simulink subsystem "harmonicFeatures"  (R2020b)
settings: Solver=VariableStepAuto  StartTime=0.0  StopTime=10.0  RelTol=1e-3
undefined symbols (not defined in the file or in its folder): params
libraries: dspstat3 x1
settings Model: Creator=trevor  LastModifiedBy=trevor

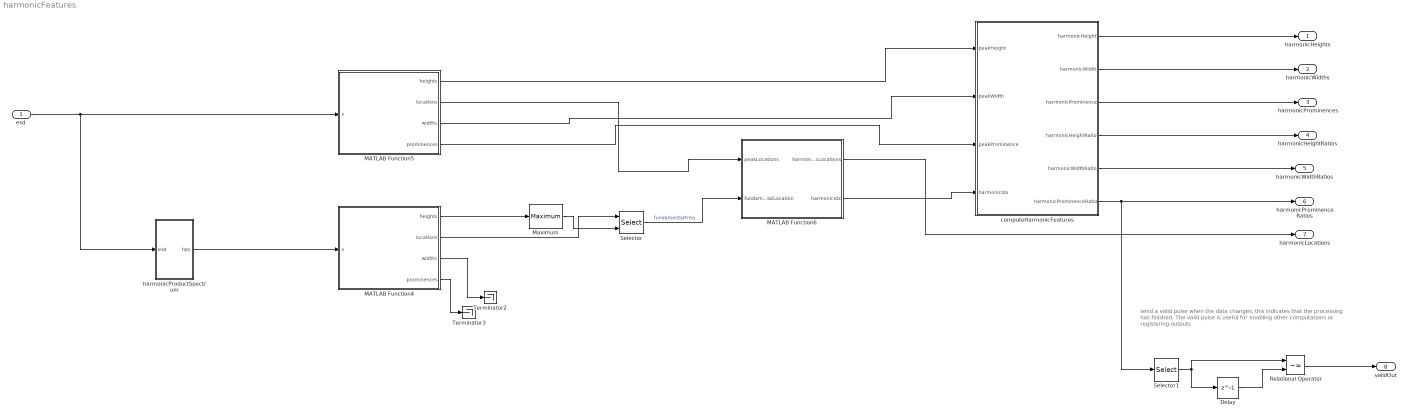
== system harmonicFeatures ==
  note: send a valid pulse when the data changes;
      | this indicates that the processing has finished.
      | The valid pulse is useful for enabling other
      | computations or registering outputs
  esd : Inport
  Delay : Delay  DelayLength=1
  MATLAB Function4 : MATLAB Function  TreatAsAtomicUnit=on
  MATLAB Function5 : MATLAB Function  TreatAsAtomicUnit=on
  MATLAB Function6 : MATLAB Function  TreatAsAtomicUnit=on
  Maximum : dspstat3/Maximum  operation=maximum  fcn=Index  indexBase=One  operateOver=Each row  Dimension=1  InputProcessing=Columns as channels (frame based)  reset=None  roiEnable=off  roiType=Rectangles  roiPortion=Entire ROI  roiOutput=Individual statistics for each ROI  roiFlag=off  roundingMode=Floor  overflowMode=off  accumDataTypeStr=Inherit: Same as product output  accumLastDataTypeStr=Inherit: Same as product output
  Relational Operator : RelationalOperator  Operator=~=  OutDataTypeStr=boolean  RndMeth=Simplest
  Selector : Selector  InputPortWidth=85  IndexOptions=Index vector (port)  Indices=[1 3]  OutputSizes=1
  Selector1 : Selector  InputPortWidth=3  IndexOptions=Index vector (dialog)  Indices=1  OutputSizes=1
  Terminator2 : Terminator
  Terminator3 : Terminator
  computeHarmonicFeatures : Subsystem
  harmonicProductSpectrum : Subsystem
  harmonicHeights : Outport
  harmonicWidths : Outport  Port=2
  harmonicProminences : Outport  Port=3
  harmonicHeightRatios : Outport  Port=4
  harmonicWidthRatios : Outport  Port=5
  harmonicProminenceRatios : Outport  Port=6
  harmonicLocations : Outport  Port=7
  validOut : Outport  Port=8
  wires:
  Selector1/1 -> Delay/1, Relational Operator/1
  Delay/1 -> Relational Operator/2
  Relational Operator/1 -> validOut/1
  Maximum/1 -> Selector/2
  MATLAB Function4/1(heights) -> Maximum/1
  harmonicProductSpectrum/1(hps) -> MATLAB Function4/1(x)
  MATLAB Function4/4(prominences) -> Terminator3/1
  MATLAB Function4/3(widths) -> Terminator2/1
  MATLAB Function4/2(locations) -> Selector/1
  esd/1 -> harmonicProductSpectrum/1(esd), MATLAB Function5/1(x)
  computeHarmonicFeatures/6(harmonicProminenceRatio) -> Selector1/1, harmonicProminenceRatios/1
  computeHarmonicFeatures/1(harmonicHeight) -> harmonicHeights/1
  computeHarmonicFeatures/2(harmonicWidth) -> harmonicWidths/1
  computeHarmonicFeatures/3(harmonicProminence) -> harmonicProminences/1
  computeHarmonicFeatures/4(harmonicHeightRatio) -> harmonicHeightRatios/1
  computeHarmonicFeatures/5(harmonicWidthRatio) -> harmonicWidthRatios/1
  MATLAB Function5/1(heights) -> computeHarmonicFeatures/1(peakHeight)
  MATLAB Function5/3(widths) -> computeHarmonicFeatures/2(peakWidth)
  MATLAB Function5/4(prominences) -> computeHarmonicFeatures/3(peakProminence)
  MATLAB Function5/2(locations) -> MATLAB Function6/1(peakLocations)
  Selector/1 -> MATLAB Function6/2(fundamentalLocation)  "fundamentalFreq"
  MATLAB Function6/1(harmonicLocations) -> harmonicLocations/1
  MATLAB Function6/2(harmonicIdx) -> computeHarmonicFeatures/4(harmonicIdx)

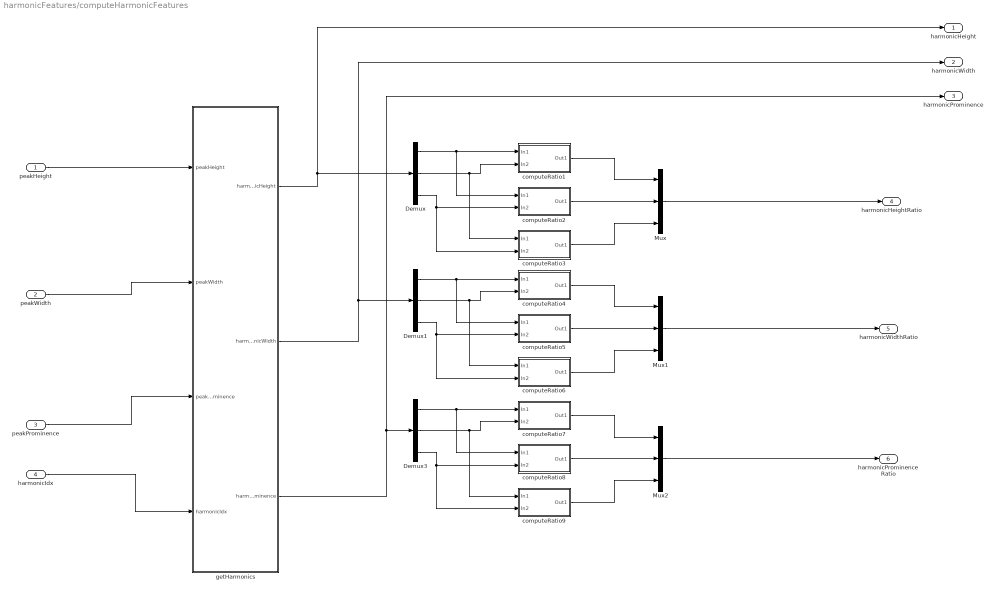
== system harmonicFeatures/computeHarmonicFeatures ==
  peakHeight : Inport
  peakWidth : Inport  Port=2
  peakProminence : Inport  Port=3
  harmonicIdx : Inport  Port=4
  Demux : Demux  Outputs=3
  Demux1 : Demux  Outputs=3
  Demux3 : Demux  Outputs=3
  Mux : Mux  Inputs=3
  Mux1 : Mux  Inputs=3
  Mux2 : Mux  Inputs=3
  computeRatio1 : Subsystem
  computeRatio2 : Subsystem
  computeRatio3 : Subsystem
  computeRatio4 : Subsystem
  computeRatio5 : Subsystem
  computeRatio6 : Subsystem
  computeRatio7 : Subsystem
  computeRatio8 : Subsystem
  computeRatio9 : Subsystem
  getHarmonics : Subsystem
  harmonicHeight : Outport
  harmonicWidth : Outport  Port=2
  harmonicProminence : Outport  Port=3
  harmonicHeightRatio : Outport  Port=4
  harmonicWidthRatio : Outport  Port=5
  harmonicProminenceRatio : Outport  Port=6
  wires:
  harmonicIdx/1 -> getHarmonics/4(harmonicIdx)
  peakProminence/1 -> getHarmonics/3(peakProminence)
  peakWidth/1 -> getHarmonics/2(peakWidth)
  peakHeight/1 -> getHarmonics/1(peakHeight)
  getHarmonics/2(harmonicWidth) -> Demux1/1, harmonicWidth/1
  getHarmonics/1(harmonicHeight) -> Demux/1, harmonicHeight/1
  getHarmonics/3(harmonicProminence) -> Demux3/1, harmonicProminence/1
  computeRatio9/1(Out1) -> Mux2/3
  computeRatio8/1(Out1) -> Mux2/2
  computeRatio7/1(Out1) -> Mux2/1
  computeRatio6/1(Out1) -> Mux1/3
  computeRatio4/1(Out1) -> Mux1/1
  computeRatio5/1(Out1) -> Mux1/2
  computeRatio3/1(Out1) -> Mux/3
  computeRatio1/1(Out1) -> Mux/1
  computeRatio2/1(Out1) -> Mux/2
  Demux3/2 -> computeRatio7/2(In2), computeRatio9/1(In1)
  Demux3/3 -> computeRatio8/2(In2), computeRatio9/2(In2)
  Demux3/1 -> computeRatio7/1(In1), computeRatio8/1(In1)
  Demux1/2 -> computeRatio4/2(In2), computeRatio6/1(In1)
  Demux1/3 -> computeRatio5/2(In2), computeRatio6/2(In2)
  Demux1/1 -> computeRatio4/1(In1), computeRatio5/1(In1)
  Demux/3 -> computeRatio2/2(In2), computeRatio3/2(In2)
  Demux/2 -> computeRatio1/2(In2), computeRatio3/1(In1)
  Demux/1 -> computeRatio1/1(In1), computeRatio2/1(In1)
  Mux/1 -> harmonicHeightRatio/1
  Mux1/1 -> harmonicWidthRatio/1
  Mux2/1 -> harmonicProminenceRatio/1

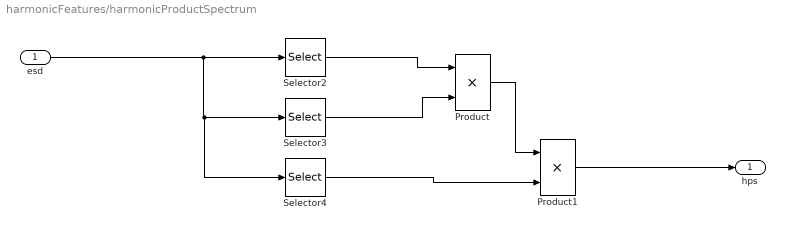
== system harmonicFeatures/harmonicProductSpectrum ==
  esd : Inport
  Product : Product  OutMin=0  OutMax=1
  Product1 : Product  OutDataTypeStr=Inherit: Same as first input
  Selector2 : Selector  InputPortWidth=512  IndexOptions=Index vector (dialog)  Indices=[1:1:170]  OutputSizes=1
  Selector3 : Selector  InputPortWidth=512  IndexOptions=Index vector (dialog)  Indices=[1:2:2*170]  OutputSizes=1
  Selector4 : Selector  InputPortWidth=512  IndexOptions=Index vector (dialog)  Indices=[1:3:3*170]  OutputSizes=1
  hps : Outport
  wires:
  Selector2/1 -> Product/1
  Product/1 -> Product1/1
  Selector4/1 -> Product1/2
  Product1/1 -> hps/1
  esd/1 -> Selector2/1, Selector3/1, Selector4/1
  Selector3/1 -> Product/2

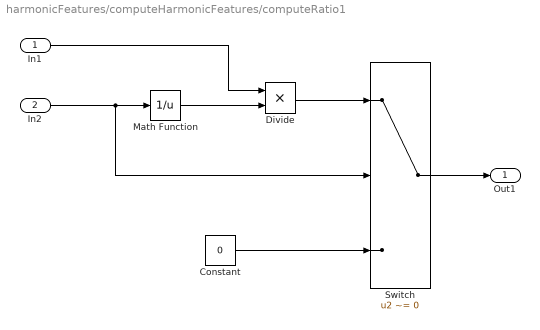
== system harmonicFeatures/computeHarmonicFeatures/computeRatio1 ==
  In1 : Inport
  In2 : Inport  Port=2
  Constant : Constant  Value=0  OutDataTypeStr=Inherit: Inherit via back propagation  SampleTime=params.systemClockPeriod
  Divide : Product  Inputs=**  OutDataTypeStr=Inherit: Keep MSB
  Math Function : Math  Operator=reciprocal  RndMeth=Zero  SaturateOnIntegerOverflow=on  OutDataTypeStr=Inherit: Inherit via internal rule
  Switch : Switch  Criteria=u2 ~= 0
  Out1 : Outport
  wires:
  Math Function/1 -> Divide/2
  Constant/1 -> Switch/3
  In2/1 -> Math Function/1, Switch/2
  Switch/1 -> Out1/1
  Divide/1 -> Switch/1
  In1/1 -> Divide/1

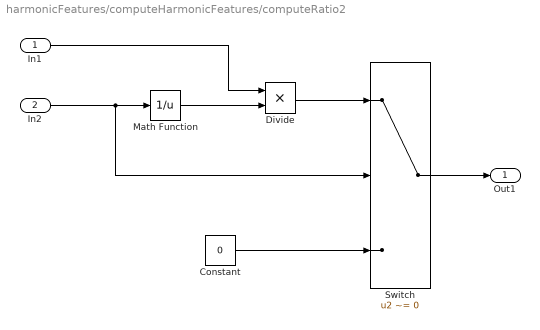
== system harmonicFeatures/computeHarmonicFeatures/computeRatio2 ==
  In1 : Inport
  In2 : Inport  Port=2
  Constant : Constant  Value=0  OutDataTypeStr=Inherit: Inherit via back propagation  SampleTime=params.systemClockPeriod
  Divide : Product  Inputs=**  OutDataTypeStr=Inherit: Keep MSB
  Math Function : Math  Operator=reciprocal  RndMeth=Zero  SaturateOnIntegerOverflow=on  OutDataTypeStr=Inherit: Inherit via internal rule
  Switch : Switch  Criteria=u2 ~= 0
  Out1 : Outport
  wires:
  Math Function/1 -> Divide/2
  Constant/1 -> Switch/3
  In2/1 -> Math Function/1, Switch/2
  Switch/1 -> Out1/1
  Divide/1 -> Switch/1
  In1/1 -> Divide/1

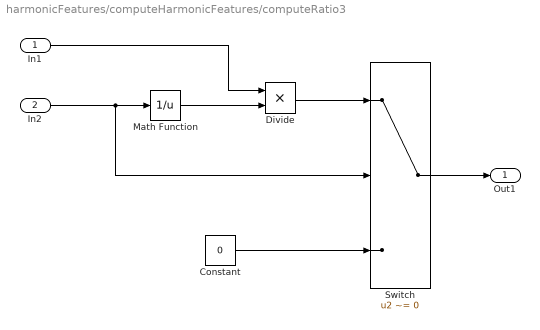
== system harmonicFeatures/computeHarmonicFeatures/computeRatio3 ==
  In1 : Inport
  In2 : Inport  Port=2
  Constant : Constant  Value=0  OutDataTypeStr=Inherit: Inherit via back propagation  SampleTime=params.systemClockPeriod
  Divide : Product  Inputs=**  OutDataTypeStr=Inherit: Keep MSB
  Math Function : Math  Operator=reciprocal  RndMeth=Zero  SaturateOnIntegerOverflow=on  OutDataTypeStr=Inherit: Inherit via internal rule
  Switch : Switch  Criteria=u2 ~= 0
  Out1 : Outport
  wires:
  Math Function/1 -> Divide/2
  Constant/1 -> Switch/3
  In2/1 -> Math Function/1, Switch/2
  Switch/1 -> Out1/1
  Divide/1 -> Switch/1
  In1/1 -> Divide/1

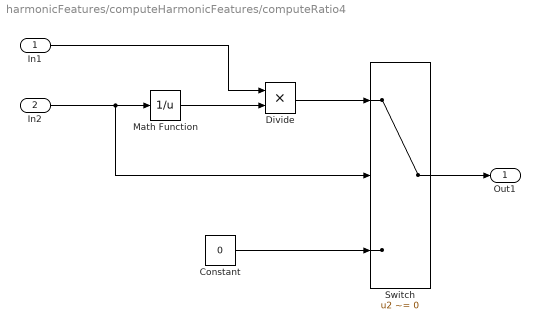
== system harmonicFeatures/computeHarmonicFeatures/computeRatio4 ==
  In1 : Inport
  In2 : Inport  Port=2
  Constant : Constant  Value=0  OutDataTypeStr=Inherit: Inherit via back propagation  SampleTime=params.systemClockPeriod
  Divide : Product  Inputs=**  OutDataTypeStr=Inherit: Keep MSB
  Math Function : Math  Operator=reciprocal  RndMeth=Zero  SaturateOnIntegerOverflow=on  OutDataTypeStr=Inherit: Inherit via internal rule
  Switch : Switch  Criteria=u2 ~= 0
  Out1 : Outport
  wires:
  Math Function/1 -> Divide/2
  Constant/1 -> Switch/3
  In2/1 -> Math Function/1, Switch/2
  Switch/1 -> Out1/1
  Divide/1 -> Switch/1
  In1/1 -> Divide/1

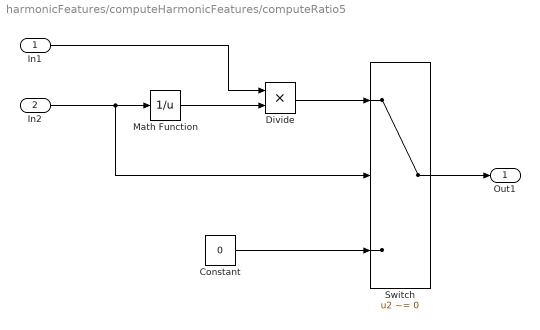
== system harmonicFeatures/computeHarmonicFeatures/computeRatio5 ==
  In1 : Inport
  In2 : Inport  Port=2
  Constant : Constant  Value=0  OutDataTypeStr=Inherit: Inherit via back propagation  SampleTime=params.systemClockPeriod
  Divide : Product  Inputs=**  OutDataTypeStr=Inherit: Keep MSB
  Math Function : Math  Operator=reciprocal  RndMeth=Zero  SaturateOnIntegerOverflow=on  OutDataTypeStr=Inherit: Inherit via internal rule
  Switch : Switch  Criteria=u2 ~= 0
  Out1 : Outport
  wires:
  Math Function/1 -> Divide/2
  Constant/1 -> Switch/3
  In2/1 -> Math Function/1, Switch/2
  Switch/1 -> Out1/1
  Divide/1 -> Switch/1
  In1/1 -> Divide/1

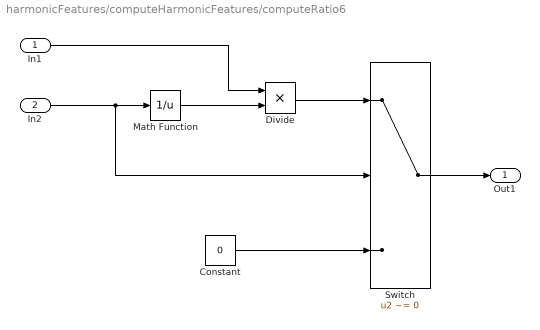
== system harmonicFeatures/computeHarmonicFeatures/computeRatio6 ==
  In1 : Inport
  In2 : Inport  Port=2
  Constant : Constant  Value=0  OutDataTypeStr=Inherit: Inherit via back propagation  SampleTime=params.systemClockPeriod
  Divide : Product  Inputs=**  OutDataTypeStr=Inherit: Keep MSB
  Math Function : Math  Operator=reciprocal  RndMeth=Zero  SaturateOnIntegerOverflow=on  OutDataTypeStr=Inherit: Inherit via internal rule
  Switch : Switch  Criteria=u2 ~= 0
  Out1 : Outport
  wires:
  Math Function/1 -> Divide/2
  Constant/1 -> Switch/3
  In2/1 -> Math Function/1, Switch/2
  Switch/1 -> Out1/1
  Divide/1 -> Switch/1
  In1/1 -> Divide/1

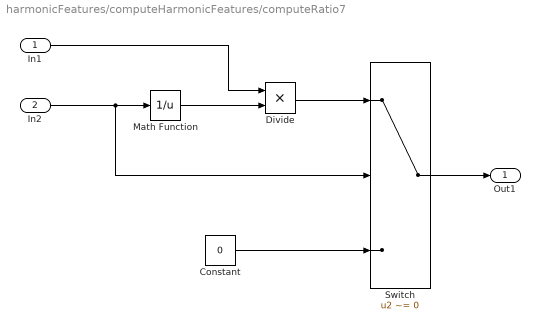
== system harmonicFeatures/computeHarmonicFeatures/computeRatio7 ==
  In1 : Inport
  In2 : Inport  Port=2
  Constant : Constant  Value=0  OutDataTypeStr=Inherit: Inherit via back propagation  SampleTime=params.systemClockPeriod
  Divide : Product  Inputs=**  OutDataTypeStr=Inherit: Keep MSB
  Math Function : Math  Operator=reciprocal  RndMeth=Zero  SaturateOnIntegerOverflow=on  OutDataTypeStr=Inherit: Inherit via internal rule
  Switch : Switch  Criteria=u2 ~= 0
  Out1 : Outport
  wires:
  Math Function/1 -> Divide/2
  Constant/1 -> Switch/3
  In2/1 -> Math Function/1, Switch/2
  Switch/1 -> Out1/1
  Divide/1 -> Switch/1
  In1/1 -> Divide/1

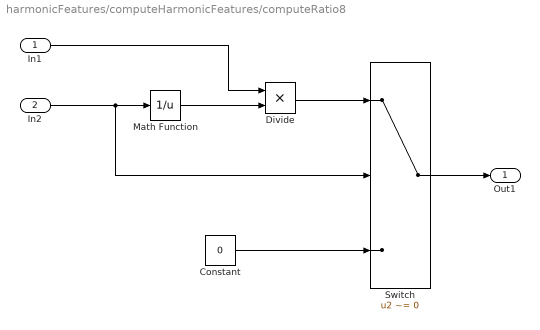
== system harmonicFeatures/computeHarmonicFeatures/computeRatio8 ==
  In1 : Inport
  In2 : Inport  Port=2
  Constant : Constant  Value=0  OutDataTypeStr=Inherit: Inherit via back propagation  SampleTime=params.systemClockPeriod
  Divide : Product  Inputs=**  OutDataTypeStr=Inherit: Keep MSB
  Math Function : Math  Operator=reciprocal  RndMeth=Zero  SaturateOnIntegerOverflow=on  OutDataTypeStr=Inherit: Inherit via internal rule
  Switch : Switch  Criteria=u2 ~= 0
  Out1 : Outport
  wires:
  Math Function/1 -> Divide/2
  Constant/1 -> Switch/3
  In2/1 -> Math Function/1, Switch/2
  Switch/1 -> Out1/1
  Divide/1 -> Switch/1
  In1/1 -> Divide/1

== system harmonicFeatures/computeHarmonicFeatures/computeRatio9 ==
  In1 : Inport
  In2 : Inport  Port=2
  Constant : Constant  Value=0  OutDataTypeStr=Inherit: Inherit via back propagation  SampleTime=params.systemClockPeriod
  Divide : Product  Inputs=**  OutDataTypeStr=Inherit: Keep MSB
  Math Function : Math  Operator=reciprocal  RndMeth=Zero  SaturateOnIntegerOverflow=on  OutDataTypeStr=Inherit: Inherit via internal rule
  Switch : Switch  Criteria=u2 ~= 0
  Out1 : Outport
  wires:
  Math Function/1 -> Divide/2
  Constant/1 -> Switch/3
  In2/1 -> Math Function/1, Switch/2
  Switch/1 -> Out1/1
  Divide/1 -> Switch/1
  In1/1 -> Divide/1

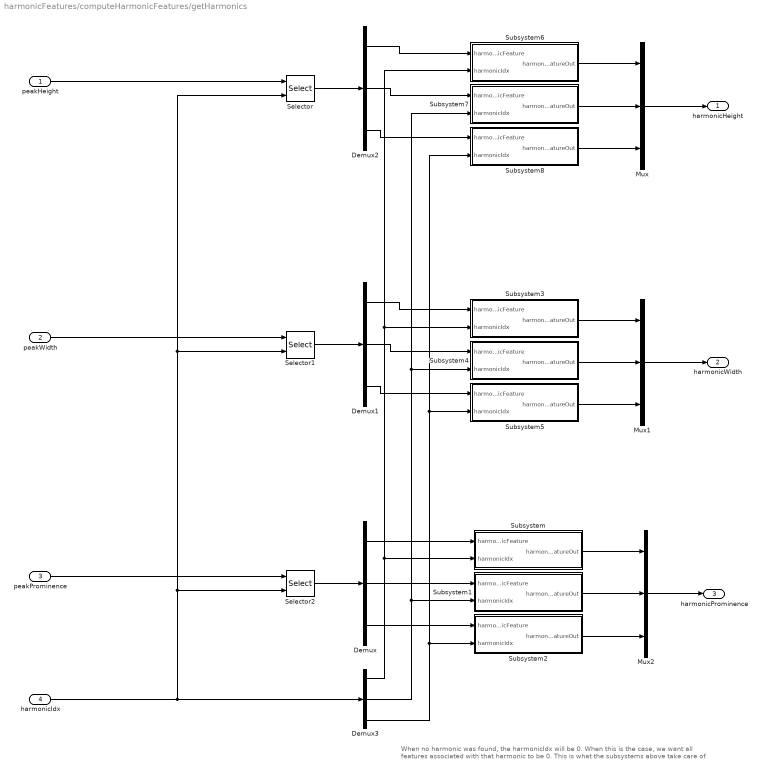
== system harmonicFeatures/computeHarmonicFeatures/getHarmonics ==
  note: When no harmonic was found, the harmonicIdx will be 0. When this is the case, we want all features associated with that harmonic to be 0. This is what the subsystems above take care of
  peakHeight : Inport
  peakWidth : Inport  Port=2
  peakProminence : Inport  Port=3
  harmonicIdx : Inport  Port=4
  Demux{,1..3} (4 alike) : Demux  Outputs=3
  Mux : Mux  Inputs=3
  Mux1 : Mux  Inputs=3
  Mux2 : Mux  Inputs=3
  Selector : Selector  InputPortWidth=256  IndexOptions=Index vector (port)  Indices=[1 3]  OutputSizes=1
  Selector1 : Selector  InputPortWidth=256  IndexOptions=Index vector (port)  Indices=[1 3]  OutputSizes=1
  Selector2 : Selector  InputPortWidth=256  IndexOptions=Index vector (port)  Indices=[1 3]  OutputSizes=1
  Subsystem : Subsystem
  Subsystem1 : Subsystem
  Subsystem2 : Subsystem
  Subsystem3 : Subsystem
  Subsystem4 : Subsystem
  Subsystem5 : Subsystem
  Subsystem6 : Subsystem
  Subsystem7 : Subsystem
  Subsystem8 : Subsystem
  harmonicHeight : Outport
  harmonicWidth : Outport  Port=2
  harmonicProminence : Outport  Port=3
  wires:
  Subsystem/1(harmonicFeatureOut) -> Mux2/1
  Subsystem1/1(harmonicFeatureOut) -> Mux2/2
  Mux2/1 -> harmonicProminence/1
  Subsystem2/1(harmonicFeatureOut) -> Mux2/3
  Subsystem3/1(harmonicFeatureOut) -> Mux1/1
  Subsystem4/1(harmonicFeatureOut) -> Mux1/2
  Mux1/1 -> harmonicWidth/1
  Subsystem5/1(harmonicFeatureOut) -> Mux1/3
  Mux/1 -> harmonicHeight/1
  Subsystem8/1(harmonicFeatureOut) -> Mux/3
  Subsystem7/1(harmonicFeatureOut) -> Mux/2
  Subsystem6/1(harmonicFeatureOut) -> Mux/1
  Demux2/2 -> Subsystem7/1(harmonicFeature)
  Demux3/1 -> Subsystem6/2(harmonicIdx), Subsystem3/2(harmonicIdx), Subsystem/2(harmonicIdx)
  Selector/1 -> Demux2/1
  Demux3/3 -> Subsystem8/2(harmonicIdx), Subsystem5/2(harmonicIdx), Subsystem2/2(harmonicIdx)
  Demux3/2 -> Subsystem7/2(harmonicIdx), Subsystem4/2(harmonicIdx), Subsystem1/2(harmonicIdx)
  Demux2/1 -> Subsystem6/1(harmonicFeature)
  Demux2/3 -> Subsystem8/1(harmonicFeature)
  Selector1/1 -> Demux1/1
  Demux1/3 -> Subsystem5/1(harmonicFeature)
  Demux1/1 -> Subsystem3/1(harmonicFeature)
  Demux1/2 -> Subsystem4/1(harmonicFeature)
  Demux/3 -> Subsystem2/1(harmonicFeature)
  Demux/2 -> Subsystem1/1(harmonicFeature)
  Demux/1 -> Subsystem/1(harmonicFeature)
  Selector2/1 -> Demux/1
  peakProminence/1 -> Selector2/1
  harmonicIdx/1 -> Demux3/1, Selector2/2, Selector/2, Selector1/2
  peakWidth/1 -> Selector1/1
  peakHeight/1 -> Selector/1

== system harmonicFeatures/computeHarmonicFeatures/getHarmonics/Subsystem ==
  harmonicFeature : Inport
  harmonicIdx : Inport  Port=2
  Constant : Constant  Value=0  OutDataTypeStr=Inherit: Inherit via back propagation  SampleTime=-1
  Switch : Switch  Criteria=u2 ~= 0
  harmonicFeatureOut : Outport
  wires:
  Constant/1 -> Switch/3
  harmonicFeature/1 -> Switch/1
  harmonicIdx/1 -> Switch/2
  Switch/1 -> harmonicFeatureOut/1

== system harmonicFeatures/computeHarmonicFeatures/getHarmonics/Subsystem1 ==
  harmonicFeature : Inport
  harmonicIdx : Inport  Port=2
  Constant : Constant  Value=0  OutDataTypeStr=Inherit: Inherit via back propagation  SampleTime=-1
  Switch : Switch  Criteria=u2 ~= 0
  harmonicFeatureOut : Outport
  wires:
  Constant/1 -> Switch/3
  harmonicFeature/1 -> Switch/1
  harmonicIdx/1 -> Switch/2
  Switch/1 -> harmonicFeatureOut/1

== system harmonicFeatures/computeHarmonicFeatures/getHarmonics/Subsystem2 ==
  harmonicFeature : Inport
  harmonicIdx : Inport  Port=2
  Constant : Constant  Value=0  OutDataTypeStr=Inherit: Inherit via back propagation  SampleTime=-1
  Switch : Switch  Criteria=u2 ~= 0
  harmonicFeatureOut : Outport
  wires:
  Constant/1 -> Switch/3
  harmonicFeature/1 -> Switch/1
  harmonicIdx/1 -> Switch/2
  Switch/1 -> harmonicFeatureOut/1

== system harmonicFeatures/computeHarmonicFeatures/getHarmonics/Subsystem3 ==
  harmonicFeature : Inport
  harmonicIdx : Inport  Port=2
  Constant : Constant  Value=0  OutDataTypeStr=Inherit: Inherit via back propagation  SampleTime=-1
  Switch : Switch  Criteria=u2 ~= 0
  harmonicFeatureOut : Outport
  wires:
  Constant/1 -> Switch/3
  harmonicFeature/1 -> Switch/1
  harmonicIdx/1 -> Switch/2
  Switch/1 -> harmonicFeatureOut/1

== system harmonicFeatures/computeHarmonicFeatures/getHarmonics/Subsystem4 ==
  harmonicFeature : Inport
  harmonicIdx : Inport  Port=2
  Constant : Constant  Value=0  OutDataTypeStr=Inherit: Inherit via back propagation  SampleTime=-1
  Switch : Switch  Criteria=u2 ~= 0
  harmonicFeatureOut : Outport
  wires:
  Constant/1 -> Switch/3
  harmonicFeature/1 -> Switch/1
  harmonicIdx/1 -> Switch/2
  Switch/1 -> harmonicFeatureOut/1

== system harmonicFeatures/computeHarmonicFeatures/getHarmonics/Subsystem5 ==
  harmonicFeature : Inport
  harmonicIdx : Inport  Port=2
  Constant : Constant  Value=0  OutDataTypeStr=Inherit: Inherit via back propagation  SampleTime=-1
  Switch : Switch  Criteria=u2 ~= 0
  harmonicFeatureOut : Outport
  wires:
  Constant/1 -> Switch/3
  harmonicFeature/1 -> Switch/1
  harmonicIdx/1 -> Switch/2
  Switch/1 -> harmonicFeatureOut/1

== system harmonicFeatures/computeHarmonicFeatures/getHarmonics/Subsystem6 ==
  harmonicFeature : Inport
  harmonicIdx : Inport  Port=2
  Constant : Constant  Value=0  OutDataTypeStr=Inherit: Inherit via back propagation  SampleTime=-1
  Switch : Switch  Criteria=u2 ~= 0
  harmonicFeatureOut : Outport
  wires:
  Constant/1 -> Switch/3
  harmonicFeature/1 -> Switch/1
  harmonicIdx/1 -> Switch/2
  Switch/1 -> harmonicFeatureOut/1

== system harmonicFeatures/computeHarmonicFeatures/getHarmonics/Subsystem7 ==
  harmonicFeature : Inport
  harmonicIdx : Inport  Port=2
  Constant : Constant  Value=0  OutDataTypeStr=Inherit: Inherit via back propagation  SampleTime=-1
  Switch : Switch  Criteria=u2 ~= 0
  harmonicFeatureOut : Outport
  wires:
  Constant/1 -> Switch/3
  harmonicFeature/1 -> Switch/1
  harmonicIdx/1 -> Switch/2
  Switch/1 -> harmonicFeatureOut/1

== system harmonicFeatures/computeHarmonicFeatures/getHarmonics/Subsystem8 ==
  harmonicFeature : Inport
  harmonicIdx : Inport  Port=2
  Constant : Constant  Value=0  OutDataTypeStr=Inherit: Inherit via back propagation  SampleTime=-1
  Switch : Switch  Criteria=u2 ~= 0
  harmonicFeatureOut : Outport
  wires:
  Constant/1 -> Switch/3
  harmonicFeature/1 -> Switch/1
  harmonicIdx/1 -> Switch/2
  Switch/1 -> harmonicFeatureOut/1

== matlab function harmonicFeatures/MATLAB Function4 ==
  settings: fimath=fimath('RoundingMethod', 'Floor','OverflowAction', 'Wrap','ProductMode', 'FullPrecision', 'SumMode', 'FullPrecision')
  data: x input; heights output; locations output; widths output; prominences output
function [heights, locations, widths, prominences] = findPeaks(x)
% findPeaks Find local maxima in a 1D signal
%
%   A peak is defined as any sample that is larger than it's neighbors.
%
%   [heights, locations, widths, prominences] = findPeaks(x) finds all peaks in
%   the signal x. It returns the height, location, width, and prominence of each
%   peak. The peak widths are measured at half-prominence height.
%
%   For plateaus, findPeaks returns the first index of the plateau.

% Much of the code contained here was ported from scipy's find_peaks
% implementation. scipy is licensed under the BSD 3-clause license.
% Copyright (c) 2001-2002 Enthought, Inc. 2003-2022, SciPy Developers
% Copyright (c) 2022 Trevor Vannoy
% SPDX-License-Identifier: BSD-3-Clause

%#codegen

locations = localMaxima1d(x);

heights = zeros(size(locations), 'like', x);
for i = 1:numel(locations)
    if locations(i) ~= 0
        heights(i) = x(locations(i));
    end
end

[prominences, leftBases, rightBases] = peakProminence(x, locations);

widths = peakWidths(x, locations, prominences, leftBases, rightBases);


end

function [locations] = localMaxima1d(x)
% localMaxima1d Find local maxima in a 1D array
%
% Inputs:
%   - x: the signal in which to find maxima
%
% Outputs:
%   - locations: the indices of each maxima/peak

% preallocate; there can't be more maxima than half the size of x
locations = zeros(1, floor(numel(x)/2), 'int16');
nPeaksIdx = uint16(1);


% the first sample can't be a maxima, so we start at 2
iMin = 2;
% last sample can't be a maxima either
iMax = numel(x) - 1;

for i =  iMin:iMax
    % if the previous sample is smaller and the next sample is at least
    % as small, we've found a peak. 
    if x(i - 1) < x(i)

        % if the next sample is equal to the current one, we've hit a plateau;
        % we return the beginning of the plateau as the peak location, which
        % is consistent with MATLAB's findpeaks behavior.
        if x(i + 1) <= x(i)
            locations(nPeaksIdx) = i;
            nPeaksIdx(:) = nPeaksIdx + 1;
        end
    end

end
end

function [prominences, leftBases, rightBases] = peakProminence(x, locations)
% peakProminence Calculate the prominence of each peak in a signal.
%
% Inputs:
%   - x: the signal
%   - locations: the locations of each peak in x
%
% Outputs:
%   - prominences: the prominence for each peak
%   - leftBases: the left base of each peak
%   - rightBases: the right base of each peak

% preallocate
prominences = zeros(size(locations), 'like', x);
leftBases = zeros(size(locations), 'like', locations);
rightBases = zeros(size(locations), 'like', locations);

iMin = cast(1, 'like', locations);
iMax = cast(numel(x), 'like', locations);

for peakNum = 1:numel(locations)
    % locations == 0 means there wasn't a peak, so skip those
    if locations(peakNum) ~= 0
        location = locations(peakNum);

        % Find the left base in interval [iMin, location]
        leftBases(peakNum) = location;
        i = location;
        leftMin = x(location);

        leftBorder = iMin;
        for i = iMin:iMax
            if i < location
                if x(i) >= x(location)
                    leftBorder = i;
                end
            end
        end
        for i = iMax:-1:iMin
            if i <= location && i >= leftBorder
                if x(i) < leftMin
                    leftMin = x(i);
                    leftBases(peakNum) = i;
                end
            end
        end

        % Find the right base in interval [location, iMax]
        rightBases(peakNum) = location;
        i = location;
        rightMin = x(location);

        rightBorder = iMax;
        for i = iMax:-1:iMin
            if i > location
                if x(i) >= x(location)
                    rightBorder = i;
                end
            end
        end
        for i = iMax:-1:iMin
            if i <= rightBorder && i >= location
                if x(i) < rightMin
                    rightMin = x(i);
                    rightBases(peakNum) = i;
                end
            end
        end

        prominences(peakNum) = x(location) - max(leftMin, rightMin);
    end
end
end

function widths = peakWidths(x, locations, prominences, leftBases, rightBases)
% peakWidths Calculate the half-prominence width of each peak
%
% Inputs:
%   - x: the signal
%   - locations: the locations of each peak in x
%   - prominences: the prominence for each peak
%   - leftBases: the left base of each peak
%   - rightBases: the right base of each peak
%
% Outputs:
%   - widths: the width for each peak

% widths are measured at half-prominence height
relHeight = 0.5;


iMin = cast(1, 'like', locations);
iMax = cast(numel(x), 'like', locations);

leftIp = cast(0,'like', x);
rightIp = cast(0, 'like', x);

widths = zeros(size(locations), 'like', leftIp);


for peakNum = 1:numel(locations)
    % locations == 0 means there wasn't a peak, so skip those
    if locations(peakNum) ~= 0
        leftBase = leftBases(peakNum);
        rightBase = rightBases(peakNum);
        location = locations(peakNum);

        height = x(location) - prominences(peakNum) * relHeight;

        % Find intersection point on left side
        leftIpTmp = iMin;
        done = false;
        for i = iMax:-1:iMin
            if i <= location && i >= leftBase
                if ~done
                    if x(i) <= height
                        done = true;
                        leftIpTmp = i;
                    end
                end
            end
        end
        
        if x(leftIpTmp) < height
            % Interpolate if true intersection height is between samples
            leftIp(:) = cast(leftIpTmp, 'like', leftIp) + (height - x(leftIpTmp)) / (x(leftIpTmp + 1) - x(leftIpTmp));
        else
            leftIp(:) = leftIpTmp;
        end

        % Find intersection point on right side
        rightIpTmp = iMax;
        done = false;
        for i = iMin:iMax
            if i >= location && i <= rightBase
                if ~done
                    if x(i) <= height
                        done = true;
                        rightIpTmp = i;
                    end
                end
            end
        end

        if x(rightIpTmp) < height
            % Interpolate if true intersection height is between samples
            rightIp(:) = cast(rightIpTmp, 'like', rightIp) - (height - x(rightIpTmp)) / (x(rightIpTmp - 1) - x(rightIpTmp));
        else
            rightIp(:) = rightIpTmp;
        end

        widths(peakNum) = rightIp - leftIp;
    end
end
end

== matlab function harmonicFeatures/MATLAB Function5 ==
  settings: fimath=fimath('RoundingMethod', 'Floor','OverflowAction', 'Wrap','ProductMode', 'FullPrecision', 'SumMode', 'FullPrecision')
  data: x input; heights output; locations output; widths output; prominences output
function [heights, locations, widths, prominences] = findPeaks(x)
% findPeaks Find local maxima in a 1D signal
%
%   A peak is defined as any sample that is larger than it's neighbors.
%
%   [heights, locations, widths, prominences] = findPeaks(x) finds all peaks in
%   the signal x. It returns the height, location, width, and prominence of each
%   peak. The peak widths are measured at half-prominence height.
%
%   For plateaus, findPeaks returns the first index of the plateau.

% Much of the code contained here was ported from scipy's find_peaks
% implementation. scipy is licensed under the BSD 3-clause license.
% Copyright (c) 2001-2002 Enthought, Inc. 2003-2022, SciPy Developers
% Copyright (c) 2022 Trevor Vannoy
% SPDX-License-Identifier: BSD-3-Clause

%#codegen

locations = localMaxima1d(x);

heights = zeros(size(locations), 'like', x);
for i = 1:numel(locations)
    if locations(i) ~= 0
        heights(i) = x(locations(i));
    end
end

[prominences, leftBases, rightBases] = peakProminence(x, locations);

widths = peakWidths(x, locations, prominences, leftBases, rightBases);


end

function [locations] = localMaxima1d(x)
% localMaxima1d Find local maxima in a 1D array
%
% Inputs:
%   - x: the signal in which to find maxima
%
% Outputs:
%   - locations: the indices of each maxima/peak

% preallocate; there can't be more maxima than half the size of x
locations = zeros(1, floor(numel(x)/2), 'int16');
nPeaksIdx = uint16(1);


% the first sample can't be a maxima, so we start at 2
iMin = 2;
% last sample can't be a maxima either
iMax = numel(x) - 1;

for i =  iMin:iMax
    % if the previous sample is smaller and the next sample is at least
    % as small, we've found a peak. 
    if x(i - 1) < x(i)

        % if the next sample is equal to the current one, we've hit a plateau;
        % we return the beginning of the plateau as the peak location, which
        % is consistent with MATLAB's findpeaks behavior.
        if x(i + 1) <= x(i)
            locations(nPeaksIdx) = i;
            nPeaksIdx(:) = nPeaksIdx + 1;
        end
    end

end
end

function [prominences, leftBases, rightBases] = peakProminence(x, locations)
% peakProminence Calculate the prominence of each peak in a signal.
%
% Inputs:
%   - x: the signal
%   - locations: the locations of each peak in x
%
% Outputs:
%   - prominences: the prominence for each peak
%   - leftBases: the left base of each peak
%   - rightBases: the right base of each peak

% preallocate
prominences = zeros(size(locations), 'like', x);
leftBases = zeros(size(locations), 'like', locations);
rightBases = zeros(size(locations), 'like', locations);

iMin = cast(1, 'like', locations);
iMax = cast(numel(x), 'like', locations);

for peakNum = 1:numel(locations)
    % locations == 0 means there wasn't a peak, so skip those
    if locations(peakNum) ~= 0
        location = locations(peakNum);

        % Find the left base in interval [iMin, location]
        leftBases(peakNum) = location;
        i = location;
        leftMin = x(location);

        leftBorder = iMin;
        for i = iMin:iMax
            if i < location
                if x(i) >= x(location)
                    leftBorder = i;
                end
            end
        end
        for i = iMax:-1:iMin
            if i <= location && i >= leftBorder
                if x(i) < leftMin
                    leftMin = x(i);
                    leftBases(peakNum) = i;
                end
            end
        end

        % Find the right base in interval [location, iMax]
        rightBases(peakNum) = location;
        i = location;
        rightMin = x(location);

        rightBorder = iMax;
        for i = iMax:-1:iMin
            if i > location
                if x(i) >= x(location)
                    rightBorder = i;
                end
            end
        end
        for i = iMax:-1:iMin
            if i <= rightBorder && i >= location
                if x(i) < rightMin
                    rightMin = x(i);
                    rightBases(peakNum) = i;
                end
            end
        end

        prominences(peakNum) = x(location) - max(leftMin, rightMin);
    end
end
end

function widths = peakWidths(x, locations, prominences, leftBases, rightBases)
% peakWidths Calculate the half-prominence width of each peak
%
% Inputs:
%   - x: the signal
%   - locations: the locations of each peak in x
%   - prominences: the prominence for each peak
%   - leftBases: the left base of each peak
%   - rightBases: the right base of each peak
%
% Outputs:
%   - widths: the width for each peak

% widths are measured at half-prominence height
relHeight = 0.5;


iMin = cast(1, 'like', locations);
iMax = cast(numel(x), 'like', locations);

leftIp = cast(0,'like', x);
rightIp = cast(0, 'like', x);

widths = zeros(size(locations), 'like', leftIp);


for peakNum = 1:numel(locations)
    % locations == 0 means there wasn't a peak, so skip those
    if locations(peakNum) ~= 0
        leftBase = leftBases(peakNum);
        rightBase = rightBases(peakNum);
        location = locations(peakNum);

        height = x(location) - prominences(peakNum) * relHeight;

        % Find intersection point on left side
        leftIpTmp = iMin;
        done = false;
        for i = iMax:-1:iMin
            if i <= location && i >= leftBase
                if ~done
                    if x(i) <= height
                        done = true;
                        leftIpTmp = i;
                    end
                end
            end
        end
        
        if x(leftIpTmp) < height
            % Interpolate if true intersection height is between samples
            leftIp(:) = cast(leftIpTmp, 'like', leftIp) + (height - x(leftIpTmp)) / (x(leftIpTmp + 1) - x(leftIpTmp));
        else
            leftIp(:) = leftIpTmp;
        end

        % Find intersection point on right side
        rightIpTmp = iMax;
        done = false;
        for i = iMin:iMax
            if i >= location && i <= rightBase
                if ~done
                    if x(i) <= height
                        done = true;
                        rightIpTmp = i;
                    end
                end
            end
        end

        if x(rightIpTmp) < height
            % Interpolate if true intersection height is between samples
            rightIp(:) = cast(rightIpTmp, 'like', rightIp) - (height - x(rightIpTmp)) / (x(rightIpTmp - 1) - x(rightIpTmp));
        else
            rightIp(:) = rightIpTmp;
        end

        widths(peakNum) = rightIp - leftIp;
    end
end
end

== matlab function harmonicFeatures/MATLAB Function6 ==
  settings: fimath=fimath('RoundingMethod', 'Floor','OverflowAction', 'Wrap','ProductMode', 'FullPrecision', 'SumMode', 'FullPrecision')
  data: peakLocations input; harmonicLocations output; harmonicIdx output; fundamentalLocation input
function [harmonicLocations, harmonicIdx] = findHarmonics(peakLocations, fundamentalLocation)

nHarmonics = 3;
nBins = 2;

harmonicLocations = zeros(nHarmonics, 1, 'like', peakLocations);
harmonicFreqs = zeros(nHarmonics, 1, 'like', peakLocations);
harmonicIdx = zeros(nHarmonics, 1, 'like', peakLocations);

% MATLAB indexing starts at one, so we need to remove 1 from the frequency
% location to get the actual frequency index/bin
fundamentalFreq = fundamentalLocation - 1;
peakFreqs = peakLocations - 1;

for i = 1:numel(peakLocations)
    for harmonicNum = 1:nHarmonics
        harmonic = fundamentalFreq * harmonicNum;

        freqDiff = abs(peakFreqs(i) - harmonic);
        if freqDiff <= nBins
            % the peak is within range of the theoretical harmonic frequency.
            if harmonicFreqs(harmonicNum) ~= 0
                % if a potential harmonic has already been found, check if the
                % new candidate is closer than the previous candidate. Keep the 
                % candidate that is closest to the theoretical harmonic.
                previousFreqDiff = abs(harmonicFreqs(harmonicNum) - harmonic);
                if freqDiff < previousFreqDiff
                    harmonicFreqs(harmonicNum) = peakFreqs(i);
                    harmonicIdx(harmonicNum) = i;
                end
            else
                % this is the first harmonic candidate we've found
                harmonicFreqs(harmonicNum) = peakFreqs(i);
                harmonicIdx(harmonicNum) = i;
            end
        end
    end
end

harmonicLocations = harmonicFreqs + 1;

% When we don't find a particular harmonic, e.g. harmonic 2 because the
% the harmonics are all odd, we want to return a 0 (or a NaN) to indicate that 
% no harmonic was found at that location.
for i = 1:nHarmonics
    if harmonicLocations(i) == 1
        harmonicLocations(i) = 0;
    end
end
